simulink model "dynamics_controlled"  (R2019a)
settings: Solver=VariableStepAuto  StartTime=0.0  StopTime=20.0  RelTol=1e-6
values from neighbouring files (symbols this model uses):
  H = [1, 1/2; 1/2, 1/3]    [main_script.m]
undefined symbols (not defined in the file or in its folder): f_fcn, fb_lin_alpha
settings Model: Creator=cosimodellasantina  LastModifiedBy=cosimodellasantina

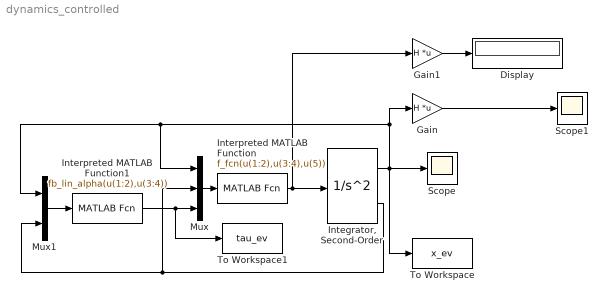
== system dynamics_controlled ==
  Display : Display
  Gain : Gain  Gain=H  Multiplication=Matrix(K*u)
  Gain1 : Gain  Gain=H  Multiplication=Matrix(K*u)
  "Integrator, Second-Order" : SecondOrderIntegrator  ICX=x_0  ICDXDT=dx_0
  Interpreted MATLAB Function : MATLABFcn  MATLABFcn=f_fcn(u(1:2),u(3:4),u(5))
  Interpreted MATLAB Function1 : MATLABFcn  MATLABFcn=fb_lin_alpha(u(1:2),u(3:4))
  Mux : Mux  Inputs=3
  Mux1 : Mux  Inputs=2
  Scope : Scope
  Scope1 : Scope
  To Workspace : ToWorkspace  VariableName=x_ev  SaveFormat=Timeseries  SampleTime=-1
  To Workspace1 : ToWorkspace  VariableName=tau_ev  SaveFormat=Timeseries  SampleTime=-1
  wires:
  "Integrator, Second-Order"/1 -> Gain/1, Mux/1, Mux1/1, To Workspace/1, Scope/1
  "Integrator, Second-Order"/2 -> Mux/2, Mux1/2
  Interpreted MATLAB Function1/1 -> To Workspace1/1, Mux/3
  Mux/1 -> Interpreted MATLAB Function/1
  Mux1/1 -> Interpreted MATLAB Function1/1
  Gain/1 -> Scope1/1
  Interpreted MATLAB Function/1 -> Gain1/1, "Integrator, Second-Order"/1
  Gain1/1 -> Display/1
